simulink library "csu_cmg_camera_geometry_lib"  (R2014b)
settings: Solver=ode45  SolverMode=SingleTasking  StartTime=0.0  StopTime=10.0  RelTol=1e-3
values from neighbouring files (symbols this model uses):
  cam_intrinsic_matrix_c = [ cam_focal_length_f/cam_pixel_size  0                                  cam_image_cx ... (first row only)    [csc_cam_camera_system_prep.m]
  cam_u_matrix = [cam_u1'/norm(cam_u1) cam_u2'/norm(cam_u2) cam_u3'/norm(cam_u3) cam_u4'/norm(cam_u4)]'    [csc_cam_camera_system_prep.m]
undefined symbols (not defined in the file or in its folder): cam_extrinsic_init, cam_image_plane_norm, cam_position_in_lander, ini_alt_wrt_1738rad
libraries: util_quat_lib x7, util_frame_rotation_lib x2, simulink x1, util_info_lib x1
settings Model: Creator=hcannon  LastModifiedBy=mstewart

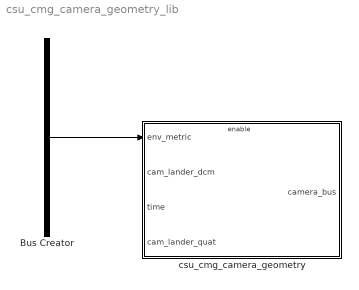
== system csu_cmg_camera_geometry_lib ==
  Bus Creator : BusCreator  Inputs=10
  csu_cmg_camera_geometry : Subsystem
  wires:
  ? -> Bus Creator/10  "grv_gravity_acc_eci"
  ? -> Bus Creator/1  "rrd_alpha_body_in_eci"
  ? -> Bus Creator/2  "rrk_rate_body_eci_body"
  ? -> Bus Creator/3  "rrk_q_body_from_eci"
  ? -> Bus Creator/4  "rrk_euler_zyx_rot_deg"
  ? -> Bus Creator/5  "rtd_acc_body_in_eci"
  ? -> Bus Creator/6  "rtk_vel_eci"
  ? -> Bus Creator/7  "rtk_pos_eci"
  ? -> Bus Creator/8
  ? -> Bus Creator/9
  Bus Creator/1 -> csu_cmg_camera_geometry/1(env_metric)

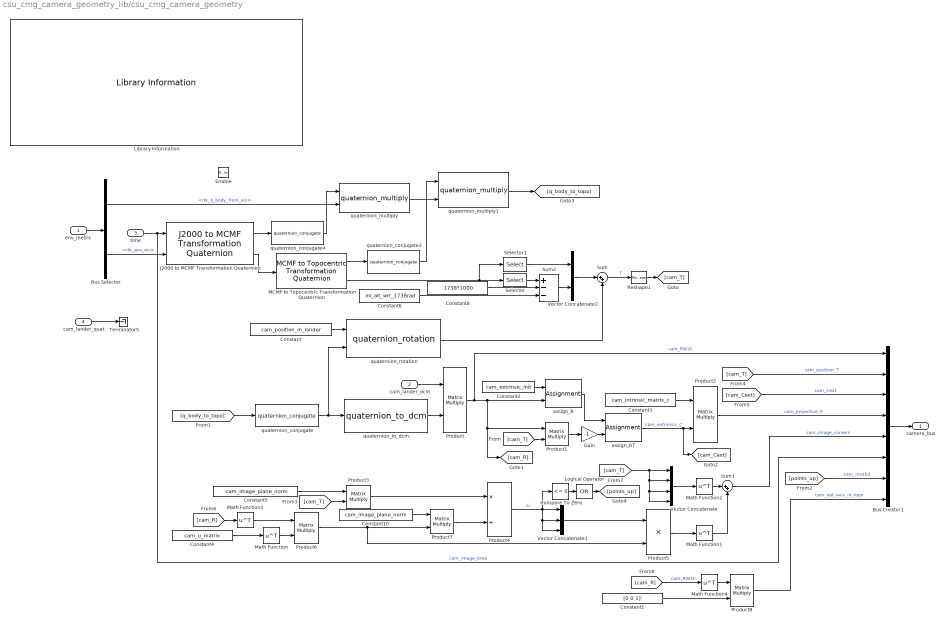
== system csu_cmg_camera_geometry_lib/csu_cmg_camera_geometry ==
  env_metric : Inport
  cam_lander_dcm : Inport  Port=2
  time : Inport  Port=3
  cam_lander_quat : Inport  Port=4
  Enable : EnablePort
  Bus Creator1 : BusCreator  Inputs=8
  Bus Selector : BusSelector  OutputSignals=lander_state_bus.rrk_q_body_from_eci,lander_state_bus.rtk_pos_eci
  Compare To Zero : simulink/Logic and Bit Operations/Compare To Zero  relop=<=  OutDataTypeStr=boolean
  Constant : Constant  Value=cam_position_in_lander
  Constant1 : Constant  Value=[0 0 1]'  VectorParams1D=off
  Constant10 : Constant  Value=cam_image_plane_norm  VectorParams1D=off
  Constant2 : Constant  Value=cam_extrinsic_init
  Constant3 : Constant  Value=cam_intrinsic_matrix_c
  Constant4 : Constant  Value=cam_u_matrix
  Constant5 : Constant  Value=-cam_image_plane_norm  VectorParams1D=off
  Constant6 : Constant  Value=ini_alt_wrt_1738rad
  Constant8 : Constant  Value=1738*1000
  Gain : Gain  Gain=-1
  J2000 to MCMF Transformation Quaternion : util_frame_rotation_lib/J2000 to MCMF  Transformation Quaternion  SystemSampleTime=-1
  Library Information : util_info_lib/Library Information  owner='NONE'
  Logical Operator : Logic  Operator=OR  Inputs=1  AllPortsSameDT=off  OutDataTypeStr=boolean
  MCMF to Topocentric Transformation Quaternion : util_frame_rotation_lib/MCMF to Topocentric  Transformation Quaternion  SystemSampleTime=-1
  Math Function{,1..4} (5 alike) : Math  Operator=transpose  SaturateOnIntegerOverflow=on
  Product{,1..3,6..8} (7 alike) : Product  Multiplication=Matrix(*)  RndMeth=Zero
  Product4 : Product  Inputs=*/  RndMeth=Zero
  Product5 : Product  Inputs=**  RndMeth=Zero
  Reshape1 : Reshape  OutputDimensionality=Column vector (2-D)
  Selector : Selector  InputPortWidth=3  Indices=[3]
  Selector1 : Selector  InputPortWidth=3  Indices=[1 2]
  Sum : Sum  Inputs=|++
  Sum1 : Sum  Inputs=|++
  Sum2 : Sum  Inputs=+--
  Terminator5 : Terminator
  Vector Concatenate : Concatenate  NumInputs=4  Mode=Multidimensional array  ConcatenateDimension=2
  Vector Concatenate1 : Concatenate  NumInputs=3  Mode=Multidimensional array
  Vector Concatenate2 : Concatenate
  assign_R : Assignment  NumberOfDimensions=2  IndexOptions=Index vector (dialog),Index vector (dialog)  Indices=[1 2 3],[1 2 3]  OutputSizes=1,1
  assign_RT : Assignment  NumberOfDimensions=2  IndexOptions=Index vector (dialog),Index vector (dialog)  Indices=[1 2 3],[4]  OutputSizes=1,1
  quaternion_conjugate : util_quat_lib/quaternion_conjugate  SystemSampleTime=-1
  quaternion_conjugate3 : util_quat_lib/quaternion_conjugate  SystemSampleTime=-1
  quaternion_conjugate4 : util_quat_lib/quaternion_conjugate  SystemSampleTime=-1
  quaternion_multiply : util_quat_lib/quaternion_multiply  SystemSampleTime=-1
  quaternion_multiply1 : util_quat_lib/quaternion_multiply  SystemSampleTime=-1
  quaternion_rotation : util_quat_lib/quaternion_rotation  SystemSampleTime=-1
  quaternion_to_dcm : util_quat_lib/quaternion_to_dcm  SystemSampleTime=-1
  camera_bus : Outport
  wires:
  Product8/1 -> Bus Creator1/8  "cam_opt_axis_in_topo"
  Constant1/1 -> Product8/2
  Math Function4/1 -> Product8/1
  [cam_R] -> Math Function4/1  "cam_RW2C"
  cam_lander_dcm/1 -> Product/1
  quaternion_to_dcm/1 -> Product/2
  time/1 -> Bus Creator1/6, J2000 to MCMF Transformation Quaternion/1  "cam_image_time"
  J2000 to MCMF Transformation Quaternion/1 -> quaternion_conjugate4/1
  quaternion_conjugate4/1 -> quaternion_multiply/1
  Bus Selector/1 -> quaternion_multiply/2  "<rrk_q_body_from_eci>"
  quaternion_multiply/1 -> quaternion_multiply1/2
  quaternion_conjugate3/1 -> quaternion_multiply1/1
  MCMF to Topocentric Transformation Quaternion/1 -> quaternion_conjugate3/1
  quaternion_conjugate/1 -> quaternion_to_dcm/1, quaternion_rotation/2
  Math Function1/1 -> Sum1/2
  Constant10/1 -> Product7/1
  [cam_T] -> Product3/2
  Constant5/1 -> Product3/1
  Math Function3/1 -> Product6/1
  quaternion_multiply1/1 -> [q_body_to_topo]
  Vector Concatenate2/1 -> Sum/1
  Sum2/1 -> Vector Concatenate2/2
  Selector/1 -> Sum2/1
  Selector1/1 -> Vector Concatenate2/1
  Constant8/1 -> Sum2/2
  Constant6/1 -> Sum2/3
  MCMF to Topocentric Transformation Quaternion/2 -> Selector1/1, Selector/1
  Reshape1/1 -> [cam_T]
  Vector Concatenate1/1 -> Product5/1
  Product4/1 -> Compare To Zero/1, Vector Concatenate1/3, Vector Concatenate1/2, Vector Concatenate1/1  "si"
  [cam_T] -> Vector Concatenate/4, Vector Concatenate/3, Vector Concatenate/2, Vector Concatenate/1
  Vector Concatenate/1 -> Math Function2/1
  Math Function2/1 -> Sum1/1
  Math Function/1 -> Product6/2
  [cam_R] -> Math Function3/1
  Constant4/1 -> Math Function/1
  Product6/1 -> Product7/2, Product5/2
  J2000 to MCMF Transformation Quaternion/2 -> MCMF to Topocentric Transformation Quaternion/1
  env_metric/1 -> Bus Selector/1
  Bus Selector/2 -> J2000 to MCMF Transformation Quaternion/2  "<rtk_pos_eci>"
  [q_body_to_topo] -> quaternion_conjugate/1
  Constant/1 -> quaternion_rotation/1
  quaternion_rotation/1 -> Sum/2
  Product/1 -> [cam_R], Product1/1, assign_R/2, Bus Creator1/1  "cam_RW2C"
  Constant2/1 -> assign_R/1
  Sum/1 -> Reshape1/1  "T"
  [cam_T] -> Product1/2
  assign_R/1 -> assign_RT/1
  Product1/1 -> Gain/1
  Gain/1 -> assign_RT/2
  assign_RT/1 -> Product2/2, [cam_Cext]  "cam_extriinsic_C"
  Product2/1 -> Bus Creator1/4  "cam_projective_P"
  Constant3/1 -> Product2/1
  Product3/1 -> Product4/1
  Product7/1 -> Product4/2
  Product5/1 -> Math Function1/1
  Sum1/1 -> Bus Creator1/5  "cam_image_corners"
  [cam_T] -> Bus Creator1/2  "cam_position_T"
  [cam_Cext] -> Bus Creator1/3  "cam_Cext"
  Bus Creator1/1 -> camera_bus/1
  Compare To Zero/1 -> Logical Operator/1
  Logical Operator/1 -> [points_up]
  [points_up] -> Bus Creator1/7  "cam_invalid"
  cam_lander_quat/1 -> Terminator5/1
